simulink model "LQR_FM"  (R2014a)
settings: Solver=ode45  StartTime=0.0  StopTime=4000  RelTol=1e-3
settings Model: Creator=Imaculada  LastModifiedBy=Imaculada

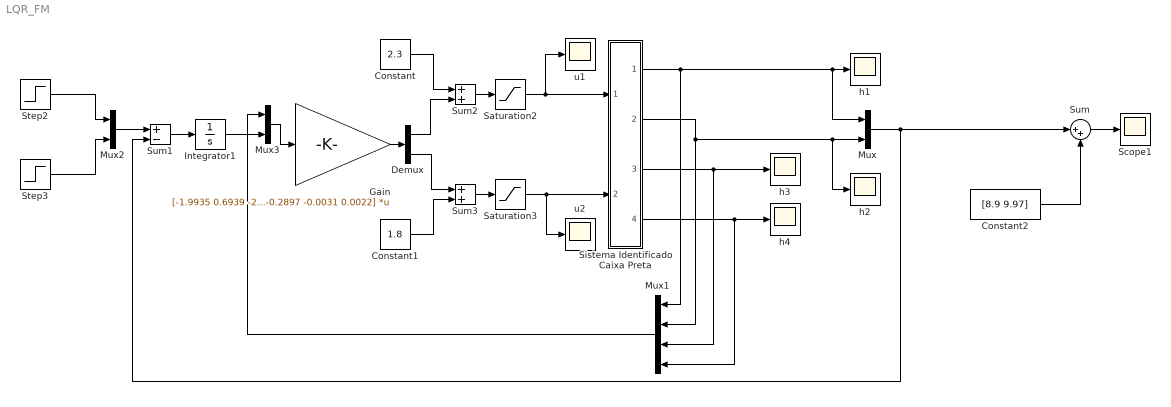
== system LQR_FM ==
  Constant : Constant  Value=2.3
  Constant1 : Constant  Value=1.8
  Constant2 : Constant  Value=[8.9 9.97]
  Demux : Demux  Outputs=2
  Gain : Gain  Gain=[-1.9935 0.6939 -2.2453 3.0809 0.0430 -0.0066 ; 0.1576 -0.1325 0.2483 -0.2897 -0.0031 0.0022]  Multiplication=Matrix(K*u)
  Integrator1 : Integrator
  Mux : Mux  Inputs=2
  Mux1 : Mux
  Mux2 : Mux  Inputs=2
  Mux3 : Mux  Inputs=2
  Saturation2 : Saturate  UpperLimit=1.5  LowerLimit=-1.5
  Saturation3 : Saturate  UpperLimit=1.5  LowerLimit=-1.5
  Scope1 : Scope
      settings: SaveName=Simulado  SampleInput=on  SampleTime=10^-1
  Sistema Identificado Caixa Preta : Subsystem
  Step2 : Step  Time=2200  SampleTime=0
  Step3 : Step  Time=2500  SampleTime=0
  Sum : Sum  Inputs=|++
  Sum1 : Sum  Inputs=+-
  Sum2 : Sum
  Sum3 : Sum
  h{1..4} (4 alike) : Scope
      h1 settings: YMin=9  YMax=17.5  SaveName=ScopeData4
      h2 settings: TimeRange=6000  SaveName=ScopeData5
      h3 settings: SaveName=ScopeData3
      h4 settings: SaveName=ScopeData6
  u1 : Scope
      settings: SaveName=ScopeData2
  u2 : Scope
  wires:
  Gain/1 -> Demux/1
  Sistema Identificado Caixa Preta/3(h3) -> Mux1/3, h3/1
  Sistema Identificado Caixa Preta/4(h4) -> Mux1/4, h4/1
  Mux/1 -> Sum/1, Sum1/2
  Mux2/1 -> Sum1/1
  Mux3/1 -> Gain/1
  Sum1/1 -> Integrator1/1
  Mux1/1 -> Mux3/1
  Demux/1 -> Sum2/2
  Step3/1 -> Mux2/2
  Step2/1 -> Mux2/1
  Integrator1/1 -> Mux3/2
  Demux/2 -> Sum3/1
  Sistema Identificado Caixa Preta/1(h1) -> h1/1, Mux/1, Mux1/1
  Sistema Identificado Caixa Preta/2(h2) -> h2/1, Mux/2, Mux1/2
  Constant1/1 -> Sum3/2
  Constant/1 -> Sum2/1
  Sum2/1 -> Saturation2/1
  Sum3/1 -> Saturation3/1
  Saturation2/1 -> Sistema Identificado Caixa Preta/1(u1), u1/1
  Saturation3/1 -> Sistema Identificado Caixa Preta/2(u2), u2/1
  Sum/1 -> Scope1/1
  Constant2/1 -> Sum/2

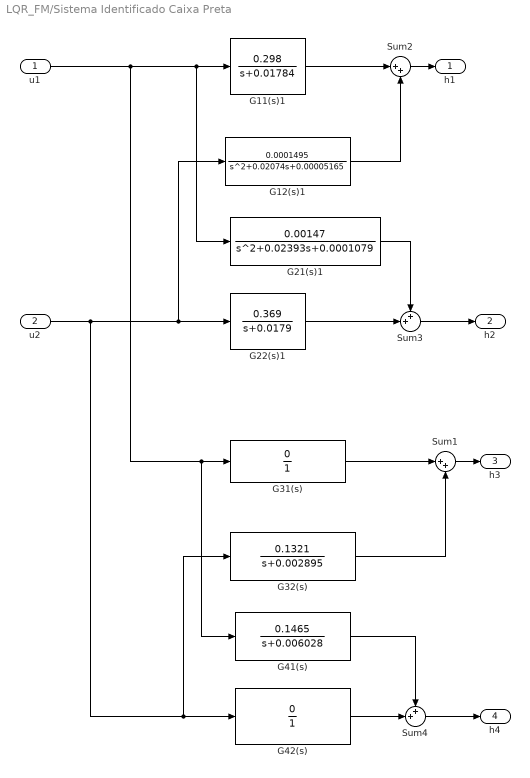
== system LQR_FM/Sistema Identificado Caixa Preta ==
  u1 : Inport
  u2 : Inport  Port=2
  G11(s)1 : TransferFcn  Numerator=[0 0.298]  Denominator=[1 0.01784]
  G12(s)1 : TransferFcn  Numerator=[0 0 0.0001495]  Denominator=[1 0.02074 0.00005165]
  G21(s)1 : TransferFcn  Numerator=[0 0 0.00147]  Denominator=[1 0.02393 0.0001079]
  G22(s)1 : TransferFcn  Numerator=[0 0.369]  Denominator=[1 0.0179]
  G31(s) : TransferFcn  Numerator=0  Denominator=1
  G32(s) : TransferFcn  Numerator=[0 0.1321]  Denominator=[1 0.002895]
  G41(s) : TransferFcn  Numerator=[0.1465]  Denominator=[1 0.006028]
  G42(s) : TransferFcn  Numerator=0  Denominator=1
  Sum1 : Sum  Inputs=|++
  Sum2 : Sum  Inputs=|++
  Sum3 : Sum  Inputs=++|
  Sum4 : Sum  Inputs=++|
  h1 : Outport
  h2 : Outport  Port=2
  h3 : Outport  Port=3
  h4 : Outport  Port=4
  wires:
  G11(s)1/1 -> Sum2/1
  G22(s)1/1 -> Sum3/2
  G12(s)1/1 -> Sum2/2
  G21(s)1/1 -> Sum3/1
  Sum2/1 -> h1/1
  Sum3/1 -> h2/1
  u1/1 -> G41(s)/1, G31(s)/1, G21(s)1/1, G11(s)1/1
  u2/1 -> G32(s)/1, G42(s)/1, G22(s)1/1, G12(s)1/1
  G31(s)/1 -> Sum1/1
  G42(s)/1 -> Sum4/2
  G32(s)/1 -> Sum1/2
  G41(s)/1 -> Sum4/1
  Sum1/1 -> h3/1
  Sum4/1 -> h4/1
